simulink model "Aufgabe4_model"  (R2020a)
settings: Solver=ode23  StartTime=0.0  StopTime=70  RelTol=1e-3
values from neighbouring files (symbols this model uses):
  A = [0, 1, 0, 0 ... (first row only)    [Aufgabe4.m]    (also in berechnung.m = simplify(subs(A)); reglerInit.m; sim_model.m)
  B = [0, -30.49, 0, 30.49]'    [Aufgabe4.m]    (also in berechnung.m = simplify(subs(B)); reglerInit.m; sim_model.m)
  C = eye(4)    [Aufgabe4.m]    (also in reglerInit.m; sim_model.m; zeitbereich_skript.m)
  Cb = [1 0 0 0 ... (first row only)    [Aufgabe4.m]    (also in reglerInit.m; sim_model.m = diag([1 0 1 0]))
  D = [0;0;0;0]    [Aufgabe4.m]    (also in reglerInit.m = [0,0,0,0]'; sim_model.m = [0,0,0,0]'; zeitbereich_skript.m = [0; 0; 0; 0])
  Kb = place(A', C', pole_beob)'    [Aufgabe4.m]    (also in reglerInit.m = place(A', Cb', pole_beob); sim_model.m = place(A', Cb', pole_beob)')
  Kz = place(A, B, pole_zustand)    [Aufgabe4.m]    (also in reglerInit.m = acker(A, B, pole_zustand))
  V = -1/(C(3,:)*inv(A-B*Kz)*B)    [Aufgabe4.m]    (also in reglerInit.m)
libraries: cstblocks x4
settings Model: Creator=jan  LastModifiedBy=jan

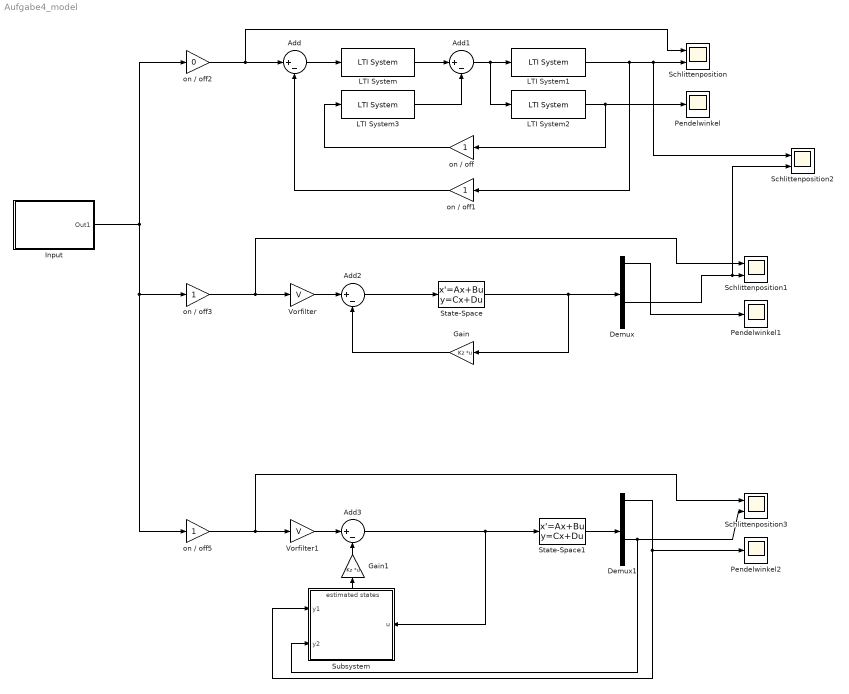
== system Aufgabe4_model ==
  Add{,1..3} (4 alike) : Sum  Inputs=|+-
  Demux : Demux
  Demux1 : Demux
  Gain : Gain  Gain=Kz  Multiplication=Matrix(K*u)
  Gain1 : Gain  Gain=Kz  Multiplication=Matrix(K*u)
  Input : Subsystem
  LTI System : cstblocks/LTI System  sys=Ks  IC=[]
  LTI System1 : cstblocks/LTI System  sys=Guy2  IC=[]
  LTI System2 : cstblocks/LTI System  sys=Guy1  IC=[]
  LTI System3 : cstblocks/LTI System  sys=Kp  IC=[]
  Pendelwinkel : Scope
  Pendelwinkel1 : Scope
  Pendelwinkel2 : Scope
  Schlittenposition{,1..3} (4 alike) : Scope  NumInputPorts=2
  State-Space : StateSpace  A=A  B=B  C=C  D=D  InitialCondition=0
  State-Space1 : StateSpace  A=A  B=B  C=C  D=D  InitialCondition=0
  Subsystem : Subsystem
      settings: PortSchema="{\"entries\":[{\"content\":{\"sides\":[{\"content\":{\"connectorIds\":[\"In1\",\"In2\"]},\"type\":\"ConnectorPlacement.EquallySpacedRectSide\",\"uuid\":\"7f2aa8f2-b163-428c-bf81-e9affbf27111\"},{\"content\":{\"connectorIds\":[\"In3\"],\"side\":\"RIGHT\"},\"type\":\"ConnectorPlacement.EquallySpacedRectSide\",\"uuid\":\"c3f9c232-c3a9-4eee-b4f1-b2439aafc6d8\"},{\"content\":{\"connectorIds\":[\"Out1\"],\"side\":\"TOP\"},\"type\":\"ConnectorPlacement.EquallySpacedRectSide\",\"uuid\":\"79f7c8b4-0d96-4164-a2ea-b62796217efe\"}]},\"type\":\"ConnectorPlacement.EquallySpacedConnector\",\"uuid\":\"ad5af13d-5e2b-4406-b284-ce2a98beb783\"}],\"packageUris\":[\"http://schema.mathworks.com/mf0/Connector/19700101\"],\"version\":\"1.0\"}"
  Vorfilter : Gain  Gain=V
  Vorfilter1 : Gain  Gain=V
  on / off{,1,3,5} (4 alike) : Gain
  on / off2 : Gain  Gain=0
  wires:
  Add/1 -> LTI System/1
  LTI System/1 -> Add1/1
  LTI System1/1 -> Schlittenposition/2, Schlittenposition2/1, on / off1/1
  Add1/1 -> LTI System2/1, LTI System1/1
  LTI System3/1 -> Add1/2
  LTI System2/1 -> Pendelwinkel/1, on / off/1
  on / off/1 -> LTI System3/1
  on / off1/1 -> Add/2
  on / off2/1 -> Schlittenposition/1, Add/1
  Gain/1 -> Add2/2
  on / off3/1 -> Vorfilter/1, Schlittenposition1/1
  Demux/3 -> Schlittenposition2/2, Schlittenposition1/2
  Vorfilter/1 -> Add2/1
  Demux/1 -> Pendelwinkel1/1
  Add2/1 -> State-Space/1
  State-Space/1 -> Gain/1, Demux/1
  on / off5/1 -> Vorfilter1/1, Schlittenposition3/1
  Input/1(Out1) -> on / off5/1, on / off3/1, on / off2/1
  Add3/1 -> Subsystem/3(u), State-Space1/1
  Demux1/1 -> Subsystem/1(y1), Pendelwinkel2/1
  State-Space1/1 -> Demux1/1
  Vorfilter1/1 -> Add3/1
  Demux1/3 -> Schlittenposition3/2, Subsystem/2(y2)
  Subsystem/1(estimated states) -> Gain1/1
  Gain1/1 -> Add3/2

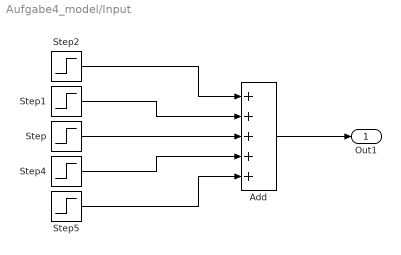
== system Aufgabe4_model/Input ==
  Add : Sum  Inputs=+++++
  Step : Step  Time=30  After=1.5  SampleTime=0
  Step1 : Step  Time=15  After=-.5  SampleTime=0
  Step2 : Step  After=.2  SampleTime=0
  Step4 : Step  Time=45  After=-.5  SampleTime=0
  Step5 : Step  Time=60  After=-.2  SampleTime=0
  Out1 : Outport
  wires:
  Add/1 -> Out1/1
  Step/1 -> Add/3
  Step4/1 -> Add/4
  Step5/1 -> Add/5
  Step1/1 -> Add/2
  Step2/1 -> Add/1

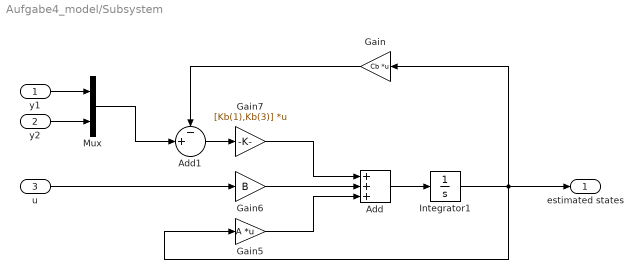
== system Aufgabe4_model/Subsystem ==
  y1 : Inport
  y2 : Inport  Port=2
  u : Inport  Port=3
  Add : Sum  Inputs=+++
  Add1 : Sum  Inputs=-+|
  Gain : Gain  Gain=Cb  Multiplication=Matrix(K*u)
  Gain5 : Gain  Gain=A  Multiplication=Matrix(K*u)
  Gain6 : Gain  Gain=B
  Gain7 : Gain  Gain=[Kb(1),Kb(3)]  Multiplication=Matrix(K*u)
  Integrator1 : Integrator
  Mux : Mux  Inputs=2
  estimated states : Outport
  wires:
  Gain7/1 -> Add/1
  Integrator1/1 -> estimated states/1, Gain/1, Gain5/1
  Add/1 -> Integrator1/1
  Mux/1 -> Add1/2
  Gain5/1 -> Add/3
  u/1 -> Gain6/1
  Gain6/1 -> Add/2
  y1/1 -> Mux/1
  y2/1 -> Mux/2
  Add1/1 -> Gain7/1
  Gain/1 -> Add1/1
